simulink library "libMdl_eulerToQuat"  (R2019b)
settings: Solver=VariableStepAuto  StartTime=0.0  StopTime=10.0  RelTol=1e-3
settings Model: Creator=hwinter  LastModifiedBy=Hanno
settings DataIOCC: ReturnWorkspaceOutputs=off
settings DebuggingCC: ArithmeticOperatorsInVariantConditions=warning
settings SFSimCC: SimUseLocalCustomCode=off  CustomCodeUndefinedFunction=UseInterfaceOnly
settings RTWCC: RTWUseLocalCustomCode=off

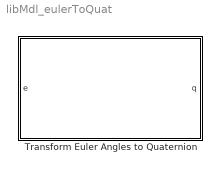
== system libMdl_eulerToQuat ==
  Transform Euler Angles to Quaternion : Subsystem
      mask Display:
      | color('black')
      | text(0.5,0.5,'Rotation order: ZYX','horizontalAlignment', 'center')

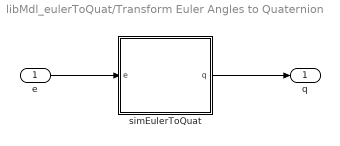
== system libMdl_eulerToQuat/Transform Euler Angles to Quaternion ==
  e : Inport
  simEulerToQuat : MATLAB Function  TreatAsAtomicUnit=on
  q : Outport  VectorParamsAs1DForOutWhenUnconnected=off
  wires:
  simEulerToQuat/1(q) -> q/1
  e/1 -> simEulerToQuat/1(e)

== matlab function libMdl_eulerToQuat/Transform Euler Angles to Quaternion/simEulerToQuat ==
  data: e input; q output
function q = simEulerToQuat(e)

q = eulerToQuat(e);

end % function
